simulink model "scars_example_control_design"  (R2019b)
settings: Solver=ode14x  StartTime=0.0  StopTime=300  FixedStep=0.01  RelTol=1e-3
libraries: scars_library x8
settings Model: Creator=asmialek  LastModifiedBy=asmialek
settings DataIOCC: ReturnWorkspaceOutputsName=scars_out

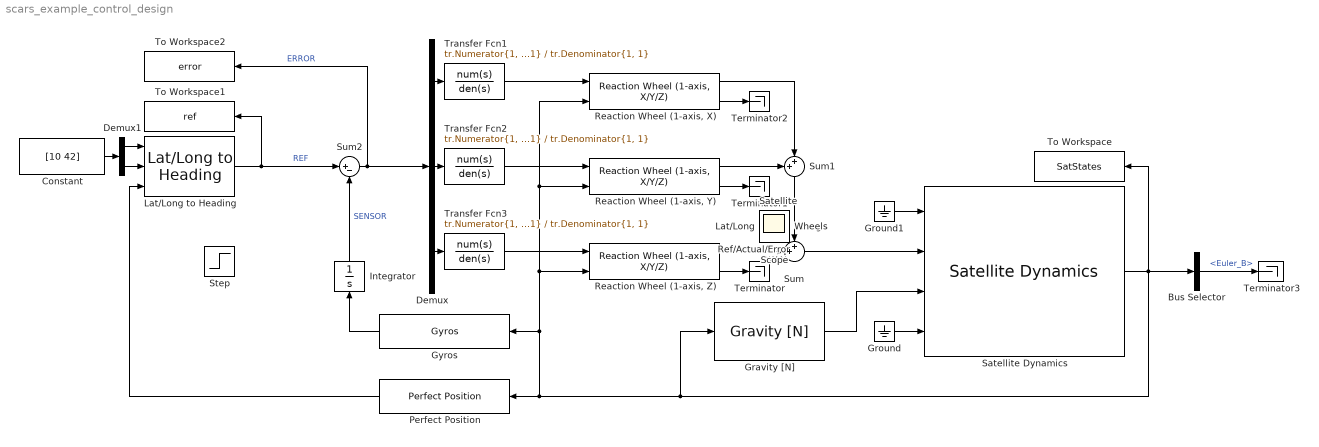
== system scars_example_control_design ==
  Bus Selector : BusSelector  OutputSignals=Euler_B
  Constant : Constant  Value=[10 42]
  Demux : Demux  Outputs=3
  Demux1 : Demux  Outputs=2
  Gravity [N] : scars_library/Environment/Gravity [N]  mass=1
  Ground : Ground
  Ground1 : Ground
  Gyros : scars_library/Sensors/Gyros  g_wn=14500  g_zeta=sqrt(2)/2  g_freq=10  g_bias=0  g_power=(2*pi*0.04/360)^2  g_max=deg2rad(75)  g_min=-deg2rad(75)
  Integrator : Integrator  InitialCondition=[0.76 2.32 1.71]
  Lat/Long to Heading : scars_library/ Control Algorithms /Lat//Long to Heading  SystemSampleTime=-1  Latency=0  AutoFrameSizeCalculation=off
  Perfect Position : scars_library/Sensors/Perfect Position  SystemSampleTime=-1  Latency=0  AutoFrameSizeCalculation=off
  "Reaction Wheel (1-axis, X)" : scars_library/Actuators/Reaction Wheel (1-axis, X//Y//Z)  axis_switch=X  N=(1.5e-3)/0.5  R=12  J=300e-3  c=0  vel_max=6000*2*pi/60  torq_max=1.5e-3  i_max=0.5  rw_power=0  rw_freq=0.1
  "Reaction Wheel (1-axis, Y)" : scars_library/Actuators/Reaction Wheel (1-axis, X//Y//Z)  axis_switch=Y  N=(1.5e-3)/0.5  R=12  J=300e-3  c=0  vel_max=6000*2*pi/60  torq_max=1.5e-3  i_max=0.5  rw_power=0  rw_freq=0.1
  "Reaction Wheel (1-axis, Z)" : scars_library/Actuators/Reaction Wheel (1-axis, X//Y//Z)  axis_switch=Z  N=(1.5e-3)/0.5  R=12  J=300e-3  c=0  vel_max=6000*2*pi/60  torq_max=1.5e-3  i_max=0.5  rw_power=0  rw_freq=0.1
  Satellite Dynamics : scars_library/Advanced/Satellite Dynamics  Parameter4=LLA Position & NED Velocity, Rotation  epoch=2451545  mass=1  a=6356e3+400e3  e=0  incl=10  RA=209.369  w=0  TA=96  initEuler=rad2deg([0.76 2.32 1.71])  initEulerRates=[0.01 0.02 0.005]  TA_copy=0  TA_copy_copy=400e3  TA_copy_copy_copy=[10 25]  TA_copy_copy_copy_copy=[1332.41761449570 7062.27056473502 -0.000303983477717348]  initEuler_copy=[0 0 0]  initEulerRates_copy=[0.01 0.02 0.005]  mask(Sattellite Dynamics){}
  Step : Step  Time=180  SampleTime=0
  Sum : Sum  Inputs=++|
  Sum1 : Sum  Inputs=++|
  Sum2 : Sum  Inputs=|+-
  Terminator{,1..3} (4 alike) : Terminator
  To Workspace : ToWorkspace  VariableName=SatStates  SaveFormat=Timeseries  SampleTime=-1
  To Workspace1 : ToWorkspace  VariableName=ref  SaveFormat=Timeseries  SampleTime=-1
  To Workspace2 : ToWorkspace  VariableName=error  SaveFormat=Timeseries  SampleTime=-1
  Transfer Fcn1 : TransferFcn  Numerator=tr.Numerator{1, 1}  Denominator=tr.Denominator{1, 1}
  Transfer Fcn2 : TransferFcn  Numerator=tr.Numerator{1, 1}  Denominator=tr.Denominator{1, 1}
  Transfer Fcn3 : TransferFcn  Numerator=tr.Numerator{1, 1}  Denominator=tr.Denominator{1, 1}
  Lat/Long : Scope
  Omega : Scope
  RW Y : Scope
  Ref/Actual/Error : Scope
  Satellite : Scope
  Scope : Scope
  Wheels : Scope
  wires:
  Ground/1 -> Satellite Dynamics/4
  Gravity [N]/1 -> Satellite Dynamics/3
  Satellite Dynamics/1 -> To Workspace/1, Bus Selector/1, Perfect Position/1, Gyros/1, "Reaction Wheel (1-axis, X)"/2, "Reaction Wheel (1-axis, Y)"/2, "Reaction Wheel (1-axis, Z)"/2, Gravity [N]/1
  Ground1/1 -> Satellite Dynamics/1
  "Reaction Wheel (1-axis, Z)"/1 -> Sum/2
  "Reaction Wheel (1-axis, Z)"/2 -> Terminator/1
  "Reaction Wheel (1-axis, Y)"/2 -> Terminator1/1
  "Reaction Wheel (1-axis, X)"/2 -> Terminator2/1
  Sum/1 -> Satellite Dynamics/2
  "Reaction Wheel (1-axis, Y)"/1 -> Sum1/1
  Sum1/1 -> Sum/1
  "Reaction Wheel (1-axis, X)"/1 -> Sum1/2
  Sum2/1 -> To Workspace2/1, Demux/1  "ERROR"
  Lat/Long to Heading/1 -> Sum2/1, To Workspace1/1  "REF"
  Gyros/1 -> Integrator/1
  Transfer Fcn1/1 -> "Reaction Wheel (1-axis, X)"/1
  Transfer Fcn2/1 -> "Reaction Wheel (1-axis, Y)"/1
  Transfer Fcn3/1 -> "Reaction Wheel (1-axis, Z)"/1
  Demux1/1 -> Lat/Long to Heading/1
  Demux1/2 -> Lat/Long to Heading/2
  Constant/1 -> Demux1/1
  Perfect Position/1 -> Lat/Long to Heading/3
  Bus Selector/1 -> Terminator3/1  "<Euler_B>"
  Demux/2 -> Transfer Fcn2/1
  Demux/1 -> Transfer Fcn1/1
  Demux/3 -> Transfer Fcn3/1
  Integrator/1 -> Sum2/2  "SENSOR"
